simulink model "general_charger_2 (Jordans MacBook.lan's conflicted copy 2013-12-22)"  (R2013a)
settings: Solver=ode45  StartTime=0  StopTime=2.5  RelTol=1e-3
PreLoadFcn:
  | Ts =5e-6;
values from neighbouring files (symbols this model uses):
  ac_volt = 169    [charger_init.m]    (also in charger_init_simpl.m)
  Cdc = 2e-3    (= 0.002)    [charger_init.m]    (also in charger_init_simpl.m)
  dcAd = dcinvexp*(eye(dcnstates) + (Ts/2)*dcAc)    [charger_init.m]    (also in charger_init_simpl.m)
  dcBd = dcinvexp*dcBc    [charger_init.m]    (also in charger_init_simpl.m)
  dcCd = dcCc*dcinvexp*Ts    [charger_init.m]    (also in charger_init_simpl.m)
  dcDd = dcCc*dcinvexp*dcBc*(Ts/2) + dcDc    [charger_init.m]    (also in charger_init_simpl.m)
  Lin = 1.5e-3    (= 0.0015)    [charger_init.m]    (also in charger_init_simpl.m = 0.001)
  P = 1.92e3    (= 1920)    [charger_init.m]    (also in charger_init_simpl.m)
  Q = 0    [charger_init.m]    (also in charger_init_simpl.m)
  ramp = (dc_volt - Vdcmin)/(acdc_ramp_end_time)    (= 202)    [charger_init.m]    (also in charger_init_simpl.m = (dc_volt - Vdcmin)/(acdc_ramp_end_time))
  switch_Ts = 5e-5    (= 5e-05)    [charger_init.m]    (also in charger_init_simpl.m)
  sys_Ts = 5e-6    (= 5e-06)    [charger_init.m]    (also in charger_init_simpl.m)
  Vdcmin = ac_volt + 10    (= 179)    [charger_init.m]    (also in charger_init_simpl.m)
  voc = 105    [charger_init.m]    (also in charger_init_simpl.m)
undefined symbols (not defined in the file or in its folder): CESR, DiscIntNeverNeededParam, Rin
undefined symbols (not defined in the file): active_power_on, Ad, Bd, Cd, dc_volt, dcdc_iki, dcdc_ikp, dcdc_on, dcdc_vki, dcdc_vkp, Dd, dq_id_ki, dq_id_kp, dq_iq_ki, dq_iq_kp, dq_vdc_ki, dq_vdc_kp, P_ki, P_kp, Q_ki, Q_kp, reactive_power_on
libraries: simulink_extras x165, powerlib x52, simulink x29, powerlib_meascontrol x6
(part 6 of 6)

== system general_charger_2 (Jordans MacBook.lan's conflicted copy 2013-12-22)/control_stage/AC//DC Control/DQ Controller/discrete low pass filter1/q rounder9 ==
  in : Inport
  Gain9 : Gain  Gain=2^-q
  Idealized ADC quantizer : simulink_extras/Additional Discrete/Idealized ADC quantizer  NumberOfConverterBits=32  Vmin=-range  Vmax=range  OutputDataType=double  OutputNegativeValues=on
  out : Outport
  wires:
  in/1 -> Idealized ADC quantizer/1
  Idealized ADC quantizer/1 -> Gain9/1
  Gain9/1 -> out/1

== system general_charger_2 (Jordans MacBook.lan's conflicted copy 2013-12-22)/control_stage/AC//DC Control/PR Controller/Source Voltage PLL/AB->DQ ==
  A : Inport
  wt : Inport  Port=2
  Add1 : Sum  Inputs=-+
  Add2 : Sum
  Delay : Delay  DelayLength=round(1/f/4/Ts)  SampleTime=Ts
  Product{1..4} (4 alike) : Product  RndMeth=Zero
  Trigonometric Function : Trigonometry
  Trigonometric Function1 : Trigonometry  Operator=cos
  D : Outport
  Q : Outport  Port=2
  wires:
  Add2/1 -> D/1  "Vd"
  Trigonometric Function/1 -> Product2/1, Product1/1
  Product1/1 -> Add2/2
  Product4/1 -> Add2/1
  wt/1 -> Trigonometric Function1/1, Trigonometric Function/1
  Delay/1 -> Product1/2, Product3/2
  Product2/1 -> Add1/1
  Product3/1 -> Add1/2
  Add1/1 -> Q/1
  A/1 -> Delay/1, Product4/1, Product2/2
  Trigonometric Function1/1 -> Product3/1, Product4/2

== system general_charger_2 (Jordans MacBook.lan's conflicted copy 2013-12-22)/control_stage/AC//DC Control/PR Controller/Source Voltage PLL/PI2 ==
  in : Inport
  Add1 : Sum
  Add2 : Sum
  Ki : Gain  Gain=ki
  Kp : Gain  Gain=kp
  Tappe : simulink/Discrete/Tapped Delay  vinit=0.0  samptime=Ts_pi  NumDelays=1  DelayOrder=Oldest  includeCurrent=off
  Ts : Gain  Gain=Ts_pi
  integral saturation : Saturate  UpperLimit=int_sat_up  LowerLimit=int_sat_low  SampleTime=Ts_pi
  pi controller saturation : Saturate  UpperLimit=pi_sat_up  LowerLimit=pi_sat_low  SampleTime=Ts_pi
  out : Outport
  wires:
  Ts/1 -> Ki/1
  in/1 -> Kp/1, Ts/1  "vdc_error"
  Add1/1 -> integral saturation/1  "vdc_int_pi"
  Kp/1 -> Add2/2  "vdc_kp_pi"
  pi controller saturation/1 -> out/1
  Tappe/1 -> Add1/1
  Add2/1 -> pi controller saturation/1  "vdc_pi"
  Ki/1 -> Add1/2
  integral saturation/1 -> Add2/1, Tappe/1

== system general_charger_2 (Jordans MacBook.lan's conflicted copy 2013-12-22)/Measurements/Power and angle calculations/AB-DQ Transform/Vab_dq/AB->DQ/Vd Discretization Error Correction ==
  A : Inport
  wt : Inport  Port=2
  D : Inport  Port=3
  Add1 : Sum  Inputs=-+
  Add2 : Sum  Inputs=-+
  Gain2 : Gain  Gain=0.000078956
  Gain3 : Gain  Gain=0.012566039
  Product : Product
  Product1 : Product
  Product2 : Product
  Trigonometric Function : Trigonometry
  Trigonometric Function1 : Trigonometry
  Trigonometric Function2 : Trigonometry
  Trigonometric Function3 : Trigonometry  Operator=cos
  Vd_corr : Outport
  wires:
  Add1/1 -> Product2/2
  Add2/1 -> Vd_corr/1
  A/1 -> Product2/1
  wt/1 -> Trigonometric Function2/1, Trigonometric Function3/1, Trigonometric Function/1, Trigonometric Function1/1
  Trigonometric Function/1 -> Product/2
  Trigonometric Function3/1 -> Product1/2
  Product1/1 -> Gain3/1
  Product2/1 -> Add2/1
  Trigonometric Function1/1 -> Product/1
  Product/1 -> Gain2/1
  D/1 -> Add2/2
  Gain3/1 -> Add1/1
  Trigonometric Function2/1 -> Product1/1
  Gain2/1 -> Add1/2

== system general_charger_2 (Jordans MacBook.lan's conflicted copy 2013-12-22)/Measurements/Power and angle calculations/AB-DQ Transform/Vab_dq/AB->DQ/Vq Discretization Error Correction ==
  Q : Inport
  wt : Inport  Port=2
  A : Inport  Port=3
  Add1 : Sum  Inputs=-+
  Add2 : Sum
  Gain2 : Gain  Gain=0.000078956
  Gain3 : Gain  Gain=-0.012566039
  Product : Product
  Product1 : Product
  Product3 : Product
  Trigonometric Function : Trigonometry  Operator=cos
  Trigonometric Function1 : Trigonometry  Operator=cos
  Trigonometric Function2 : Trigonometry
  Trigonometric Function3 : Trigonometry  Operator=cos
  Vq_corr : Outport
  wires:
  wt/1 -> Trigonometric Function2/1, Trigonometric Function/1, Trigonometric Function1/1, Trigonometric Function3/1
  Trigonometric Function2/1 -> Product1/1
  Trigonometric Function3/1 -> Product1/2
  Product1/1 -> Gain2/1
  Trigonometric Function1/1 -> Product3/1
  Trigonometric Function/1 -> Product3/2
  Product3/1 -> Gain3/1
  Gain2/1 -> Add2/1
  Gain3/1 -> Add2/2
  Add2/1 -> Product/2
  A/1 -> Product/1
  Product/1 -> Add1/1
  Q/1 -> Add1/2
  Add1/1 -> Vq_corr/1

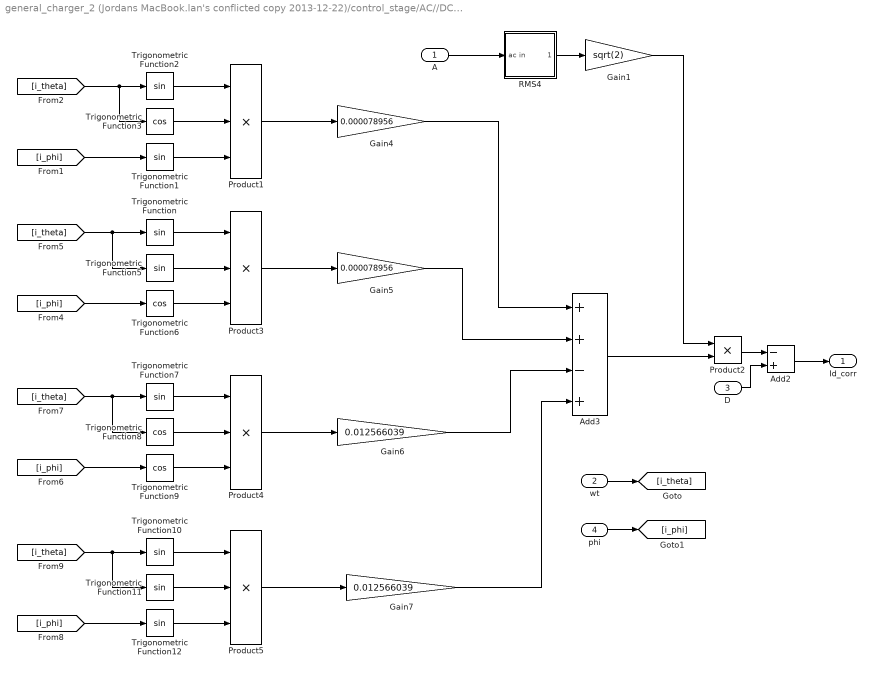
== system general_charger_2 (Jordans MacBook.lan's conflicted copy 2013-12-22)/control_stage/AC//DC Control/DQ Controller/AB-DQ Transform/AB->DQ/Id Discretization Error Correction ==
  A : Inport
  wt : Inport  Port=2
  D : Inport  Port=3
  phi : Inport  Port=4
  Add2 : Sum  Inputs=-+
  Add3 : Sum  Inputs=++-+
  Gain1 : Gain  Gain=sqrt(2)
  Gain4 : Gain  Gain=0.000078956
  Gain5 : Gain  Gain=0.000078956
  Gain6 : Gain  Gain=0.012566039
  Gain7 : Gain  Gain=0.012566039
  Product{1,3..5} (4 alike) : Product  Inputs=3
  Product2 : Product
  RMS4 : Subsystem  mask{f=60, rms_Ts=4e-4}
      mask prompts: f "Fundamental Frequency"; rms_Ts "Sample Time"
      mask init:
      | SpC=1/f/rms_Ts;
      | RSpC=ceil(SpC);
      | Delay=RSpC*rms_Ts;
      | Corr1=(SpC-RSpC)/2;
      | Corr2=(SpC-RSpC)/SpC;
      | K1=Corr1*Corr2;
      | K2=Corr2 + Corr1*Corr2;
      mask Display: disp('RMS')
  Trigonometric Function{,1..2,5,7,10..12} (8 alike) : Trigonometry
  Trigonometric Function{3,6,8..9} (4 alike) : Trigonometry  Operator=cos
  Id_corr : Outport
  wires:
  Add2/1 -> Id_corr/1
  Product2/1 -> Add2/1
  D/1 -> Add2/2
  wt/1 -> [i_theta]
  phi/1 -> [i_phi]
  [i_theta] -> Trigonometric Function3/1, Trigonometric Function2/1
  [i_phi] -> Trigonometric Function1/1
  Trigonometric Function1/1 -> Product1/3
  Trigonometric Function2/1 -> Product1/1
  Trigonometric Function3/1 -> Product1/2
  Product1/1 -> Gain4/1
  [i_theta] -> Trigonometric Function5/1, Trigonometric Function/1
  [i_phi] -> Trigonometric Function6/1
  Trigonometric Function5/1 -> Product3/2
  Trigonometric Function/1 -> Product3/1
  Trigonometric Function6/1 -> Product3/3
  [i_theta] -> Trigonometric Function8/1, Trigonometric Function7/1
  [i_phi] -> Trigonometric Function9/1
  Trigonometric Function8/1 -> Product4/2
  Trigonometric Function7/1 -> Product4/1
  Trigonometric Function9/1 -> Product4/3
  [i_theta] -> Trigonometric Function11/1, Trigonometric Function10/1
  [i_phi] -> Trigonometric Function12/1
  Trigonometric Function11/1 -> Product5/2
  Trigonometric Function10/1 -> Product5/1
  Trigonometric Function12/1 -> Product5/3
  Product3/1 -> Gain5/1
  Product4/1 -> Gain6/1
  Product5/1 -> Gain7/1
  Gain4/1 -> Add3/1
  Gain5/1 -> Add3/2
  Gain6/1 -> Add3/3
  Gain7/1 -> Add3/4
  Add3/1 -> Product2/2
  Gain1/1 -> Product2/1
  RMS4/1(rms out) -> Gain1/1
  A/1 -> RMS4/1(ac in)

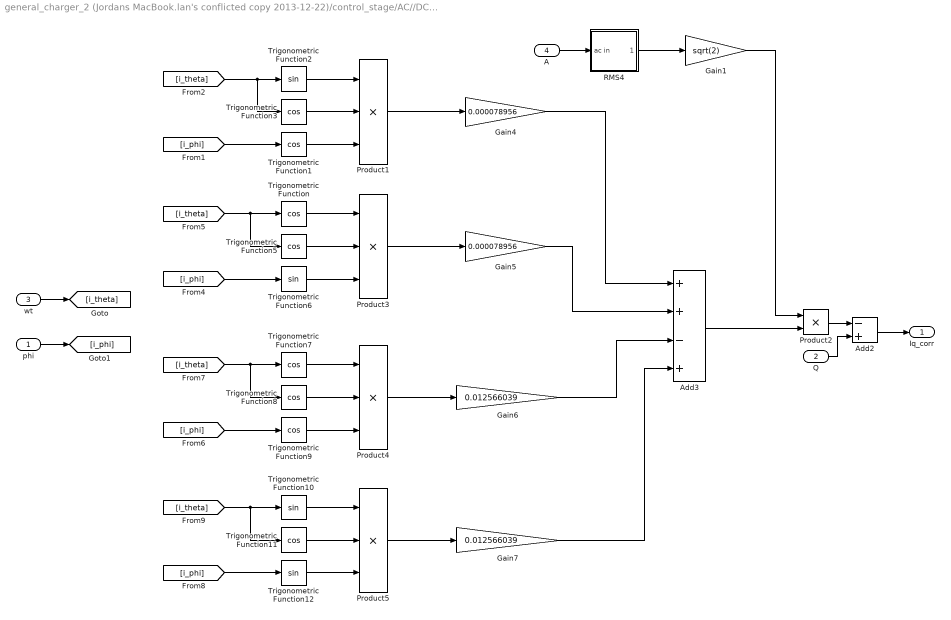
== system general_charger_2 (Jordans MacBook.lan's conflicted copy 2013-12-22)/control_stage/AC//DC Control/DQ Controller/AB-DQ Transform/AB->DQ/Iq Discretization Error Correction ==
  phi : Inport
  Q : Inport  Port=2
  wt : Inport  Port=3
  A : Inport  Port=4
  Add2 : Sum  Inputs=-+
  Add3 : Sum  Inputs=++-+
  Gain1 : Gain  Gain=sqrt(2)
  Gain4 : Gain  Gain=0.000078956
  Gain5 : Gain  Gain=0.000078956
  Gain6 : Gain  Gain=0.012566039
  Gain7 : Gain  Gain=0.012566039
  Product{1,3..5} (4 alike) : Product  Inputs=3
  Product2 : Product
  RMS4 : Subsystem  mask{f=60, rms_Ts=4e-4}
      mask prompts: f "Fundamental Frequency"; rms_Ts "Sample Time"
      mask init:
      | SpC=1/f/rms_Ts;
      | RSpC=ceil(SpC);
      | Delay=RSpC*rms_Ts;
      | Corr1=(SpC-RSpC)/2;
      | Corr2=(SpC-RSpC)/SpC;
      | K1=Corr1*Corr2;
      | K2=Corr2 + Corr1*Corr2;
      mask Display: disp('RMS')
  Trigonometric Function{,1,3,5,7..9,11} (8 alike) : Trigonometry  Operator=cos
  Trigonometric Function{2,6,10,12} (4 alike) : Trigonometry
  Iq_corr : Outport
  wires:
  Add2/1 -> Iq_corr/1
  Product2/1 -> Add2/1
  Q/1 -> Add2/2
  [i_theta] -> Trigonometric Function3/1, Trigonometric Function2/1
  [i_phi] -> Trigonometric Function1/1
  Trigonometric Function1/1 -> Product1/3
  Trigonometric Function2/1 -> Product1/1
  Trigonometric Function3/1 -> Product1/2
  Product1/1 -> Gain4/1
  [i_theta] -> Trigonometric Function5/1, Trigonometric Function/1
  [i_phi] -> Trigonometric Function6/1
  Trigonometric Function5/1 -> Product3/2
  Trigonometric Function/1 -> Product3/1
  Trigonometric Function6/1 -> Product3/3
  [i_theta] -> Trigonometric Function8/1, Trigonometric Function7/1
  [i_phi] -> Trigonometric Function9/1
  Trigonometric Function8/1 -> Product4/2
  Trigonometric Function7/1 -> Product4/1
  Trigonometric Function9/1 -> Product4/3
  [i_theta] -> Trigonometric Function11/1, Trigonometric Function10/1
  [i_phi] -> Trigonometric Function12/1
  Trigonometric Function11/1 -> Product5/2
  Trigonometric Function10/1 -> Product5/1
  Trigonometric Function12/1 -> Product5/3
  Product3/1 -> Gain5/1
  Product4/1 -> Gain6/1
  Product5/1 -> Gain7/1
  Gain4/1 -> Add3/1
  Gain5/1 -> Add3/2
  Gain6/1 -> Add3/3
  Gain7/1 -> Add3/4
  Add3/1 -> Product2/2
  Gain1/1 -> Product2/1
  wt/1 -> [i_theta]
  phi/1 -> [i_phi]
  RMS4/1(rms out) -> Gain1/1
  A/1 -> RMS4/1(ac in)

== system general_charger_2 (Jordans MacBook.lan's conflicted copy 2013-12-22)/control_stage/AC//DC Control/DQ Controller/AB-DQ Transform/PLL/AB->DQ ==
  A : Inport
  wt : Inport  Port=2
  Add1 : Sum  Inputs=-+
  Add2 : Sum
  Delay : Delay  DelayLength=RSpC  SampleTime=abdq_Ts
  Product{1..4} (4 alike) : Product  RndMeth=Zero
  Trigonometric Function : Trigonometry
  Trigonometric Function1 : Trigonometry  Operator=cos
  Vd Discretization Error Correction : Subsystem
  Vq Discretization Error Correction : Subsystem
  D : Outport
  Q : Outport  Port=2
  wires:
  Trigonometric Function/1 -> Product1/1, Product2/1
  Product1/1 -> Add2/2
  Product4/1 -> Add2/1
  Product2/1 -> Add1/1
  A/1 -> Vq Discretization Error Correction/3(A), Delay/1, Vd Discretization Error Correction/1(A), Product4/1, Product2/2
  Trigonometric Function1/1 -> Product4/2, Product3/1
  Product3/1 -> Add1/2
  Delay/1 -> Product1/2, Product3/2  "B"
  wt/1 -> [theta], Trigonometric Function1/1, Trigonometric Function/1
  Add2/1 -> Vd Discretization Error Correction/3(D)  "Vd"
  Add1/1 -> Vq Discretization Error Correction/1(Q)
  [theta] -> Vq Discretization Error Correction/2(wt)
  [theta] -> Vd Discretization Error Correction/2(wt)
  Vd Discretization Error Correction/1(Vd_corr) -> D/1
  Vq Discretization Error Correction/1(Vq_corr) -> Q/1

== system general_charger_2 (Jordans MacBook.lan's conflicted copy 2013-12-22)/control_stage/AC//DC Control/DQ Controller/AB-DQ Transform/PLL/PI1 ==
  in : Inport
  Add1 : Sum
  Add2 : Sum
  Ki : Gain  Gain=ki
  Kp : Gain  Gain=kp
  Tappe : simulink/Discrete/Tapped Delay  vinit=0.0  samptime=Ts_pi  NumDelays=1  DelayOrder=Oldest  includeCurrent=off
  Ts : Gain  Gain=Ts_pi
  integral saturation : Saturate  UpperLimit=int_sat_up  LowerLimit=int_sat_low  SampleTime=Ts_pi
  pi controller saturation : Saturate  UpperLimit=pi_sat_up  LowerLimit=pi_sat_low  SampleTime=Ts_pi
  out : Outport
  wires:
  Ts/1 -> Ki/1
  in/1 -> Kp/1, Ts/1  "vdc_error"
  Add1/1 -> integral saturation/1  "vdc_int_pi"
  Kp/1 -> Add2/2  "vdc_kp_pi"
  pi controller saturation/1 -> out/1
  Tappe/1 -> Add1/1
  Add2/1 -> pi controller saturation/1  "vdc_pi"
  Ki/1 -> Add1/2
  integral saturation/1 -> Add2/1, Tappe/1

== system general_charger_2 (Jordans MacBook.lan's conflicted copy 2013-12-22)/control_stage/AC//DC Control/DQ Controller/AB-DQ Transform/PLL/PI4 ==
  in : Inport
  Add1 : Sum
  Add2 : Sum
  Ki : Gain  Gain=ki
  Kp : Gain  Gain=kp
  Tappe : simulink/Discrete/Tapped Delay  vinit=0.0  samptime=Ts_pi  NumDelays=1  DelayOrder=Oldest  includeCurrent=off
  Ts : Gain  Gain=Ts_pi
  integral saturation : Saturate  UpperLimit=int_sat_up  LowerLimit=int_sat_low  SampleTime=Ts_pi
  pi controller saturation : Saturate  UpperLimit=pi_sat_up  LowerLimit=pi_sat_low  SampleTime=Ts_pi
  out : Outport
  wires:
  Ts/1 -> Ki/1
  in/1 -> Kp/1, Ts/1  "vdc_error"
  Add1/1 -> integral saturation/1  "vdc_int_pi"
  Kp/1 -> Add2/2  "vdc_kp_pi"
  pi controller saturation/1 -> out/1
  Tappe/1 -> Add1/1
  Add2/1 -> pi controller saturation/1  "vdc_pi"
  Ki/1 -> Add1/2
  integral saturation/1 -> Add2/1, Tappe/1

== system general_charger_2 (Jordans MacBook.lan's conflicted copy 2013-12-22)/control_stage/AC//DC Control/DQ Controller/DQ Controller Submodule/Reactive Power Control Module/PI4 ==
  in : Inport
  Add1 : Sum
  Add2 : Sum
  Ki : Gain  Gain=ki
  Kp : Gain  Gain=kp
  Tappe : simulink/Discrete/Tapped Delay  vinit=0.0  samptime=Ts_pi  NumDelays=1  DelayOrder=Oldest  includeCurrent=off
  Ts : Gain  Gain=Ts_pi
  integral saturation : Saturate  UpperLimit=int_sat_up  LowerLimit=int_sat_low  SampleTime=Ts_pi
  pi controller saturation : Saturate  UpperLimit=pi_sat_up  LowerLimit=pi_sat_low  SampleTime=Ts_pi
  out : Outport
  wires:
  Ts/1 -> Ki/1
  in/1 -> Kp/1, Ts/1  "vdc_error"
  Add1/1 -> integral saturation/1  "vdc_int_pi"
  Kp/1 -> Add2/2  "vdc_kp_pi"
  pi controller saturation/1 -> out/1
  Tappe/1 -> Add1/1
  Add2/1 -> pi controller saturation/1  "vdc_pi"
  Ki/1 -> Add1/2
  integral saturation/1 -> Add2/1, Tappe/1

== system general_charger_2 (Jordans MacBook.lan's conflicted copy 2013-12-22)/control_stage/AC//DC Control/DQ Controller/discrete low pass filter1/Ad(1,1)/q rounder16 ==
  in : Inport
  Gain9 : Gain  Gain=2^-q
  Idealized ADC quantizer : simulink_extras/Additional Discrete/Idealized ADC quantizer  NumberOfConverterBits=32  Vmin=-range  Vmax=range  OutputDataType=double  OutputNegativeValues=on
  out : Outport
  wires:
  in/1 -> Idealized ADC quantizer/1
  Idealized ADC quantizer/1 -> Gain9/1
  Gain9/1 -> out/1

== system general_charger_2 (Jordans MacBook.lan's conflicted copy 2013-12-22)/control_stage/AC//DC Control/DQ Controller/discrete low pass filter1/Ad(1,2)/q rounder16 ==
  in : Inport
  Gain9 : Gain  Gain=2^-q
  Idealized ADC quantizer : simulink_extras/Additional Discrete/Idealized ADC quantizer  NumberOfConverterBits=32  Vmin=-range  Vmax=range  OutputDataType=double  OutputNegativeValues=on
  out : Outport
  wires:
  in/1 -> Idealized ADC quantizer/1
  Idealized ADC quantizer/1 -> Gain9/1
  Gain9/1 -> out/1

== system general_charger_2 (Jordans MacBook.lan's conflicted copy 2013-12-22)/control_stage/AC//DC Control/DQ Controller/discrete low pass filter1/Ad(1,3)/q rounder16 ==
  in : Inport
  Gain9 : Gain  Gain=2^-q
  Idealized ADC quantizer : simulink_extras/Additional Discrete/Idealized ADC quantizer  NumberOfConverterBits=32  Vmin=-range  Vmax=range  OutputDataType=double  OutputNegativeValues=on
  out : Outport
  wires:
  in/1 -> Idealized ADC quantizer/1
  Idealized ADC quantizer/1 -> Gain9/1
  Gain9/1 -> out/1

== system general_charger_2 (Jordans MacBook.lan's conflicted copy 2013-12-22)/control_stage/AC//DC Control/DQ Controller/discrete low pass filter1/Ad(2,1)/q rounder16 ==
  in : Inport
  Gain9 : Gain  Gain=2^-q
  Idealized ADC quantizer : simulink_extras/Additional Discrete/Idealized ADC quantizer  NumberOfConverterBits=32  Vmin=-range  Vmax=range  OutputDataType=double  OutputNegativeValues=on
  out : Outport
  wires:
  in/1 -> Idealized ADC quantizer/1
  Idealized ADC quantizer/1 -> Gain9/1
  Gain9/1 -> out/1

== system general_charger_2 (Jordans MacBook.lan's conflicted copy 2013-12-22)/control_stage/AC//DC Control/DQ Controller/discrete low pass filter1/Ad(2,2)/q rounder16 ==
  in : Inport
  Gain9 : Gain  Gain=2^-q
  Idealized ADC quantizer : simulink_extras/Additional Discrete/Idealized ADC quantizer  NumberOfConverterBits=32  Vmin=-range  Vmax=range  OutputDataType=double  OutputNegativeValues=on
  out : Outport
  wires:
  in/1 -> Idealized ADC quantizer/1
  Idealized ADC quantizer/1 -> Gain9/1
  Gain9/1 -> out/1

== system general_charger_2 (Jordans MacBook.lan's conflicted copy 2013-12-22)/control_stage/AC//DC Control/DQ Controller/discrete low pass filter1/Ad(2,3)/q rounder16 ==
  in : Inport
  Gain9 : Gain  Gain=2^-q
  Idealized ADC quantizer : simulink_extras/Additional Discrete/Idealized ADC quantizer  NumberOfConverterBits=32  Vmin=-range  Vmax=range  OutputDataType=double  OutputNegativeValues=on
  out : Outport
  wires:
  in/1 -> Idealized ADC quantizer/1
  Idealized ADC quantizer/1 -> Gain9/1
  Gain9/1 -> out/1

== system general_charger_2 (Jordans MacBook.lan's conflicted copy 2013-12-22)/control_stage/AC//DC Control/DQ Controller/discrete low pass filter1/Ad(3,1)/q rounder16 ==
  in : Inport
  Gain9 : Gain  Gain=2^-q
  Idealized ADC quantizer : simulink_extras/Additional Discrete/Idealized ADC quantizer  NumberOfConverterBits=32  Vmin=-range  Vmax=range  OutputDataType=double  OutputNegativeValues=on
  out : Outport
  wires:
  in/1 -> Idealized ADC quantizer/1
  Idealized ADC quantizer/1 -> Gain9/1
  Gain9/1 -> out/1

== system general_charger_2 (Jordans MacBook.lan's conflicted copy 2013-12-22)/control_stage/AC//DC Control/DQ Controller/discrete low pass filter1/Ad(3,2)/q rounder16 ==
  in : Inport
  Gain9 : Gain  Gain=2^-q
  Idealized ADC quantizer : simulink_extras/Additional Discrete/Idealized ADC quantizer  NumberOfConverterBits=32  Vmin=-range  Vmax=range  OutputDataType=double  OutputNegativeValues=on
  out : Outport
  wires:
  in/1 -> Idealized ADC quantizer/1
  Idealized ADC quantizer/1 -> Gain9/1
  Gain9/1 -> out/1

== system general_charger_2 (Jordans MacBook.lan's conflicted copy 2013-12-22)/control_stage/AC//DC Control/DQ Controller/discrete low pass filter1/Ad(3,3)/q rounder16 ==
  in : Inport
  Gain9 : Gain  Gain=2^-q
  Idealized ADC quantizer : simulink_extras/Additional Discrete/Idealized ADC quantizer  NumberOfConverterBits=32  Vmin=-range  Vmax=range  OutputDataType=double  OutputNegativeValues=on
  out : Outport
  wires:
  in/1 -> Idealized ADC quantizer/1
  Idealized ADC quantizer/1 -> Gain9/1
  Gain9/1 -> out/1

== system general_charger_2 (Jordans MacBook.lan's conflicted copy 2013-12-22)/control_stage/AC//DC Control/DQ Controller/discrete low pass filter1/Bd(1)/q rounder16 ==
  in : Inport
  Gain9 : Gain  Gain=2^-q
  Idealized ADC quantizer : simulink_extras/Additional Discrete/Idealized ADC quantizer  NumberOfConverterBits=32  Vmin=-range  Vmax=range  OutputDataType=double  OutputNegativeValues=on
  out : Outport
  wires:
  in/1 -> Idealized ADC quantizer/1
  Idealized ADC quantizer/1 -> Gain9/1
  Gain9/1 -> out/1

== system general_charger_2 (Jordans MacBook.lan's conflicted copy 2013-12-22)/control_stage/AC//DC Control/DQ Controller/discrete low pass filter1/Bd(2)/q rounder16 ==
  in : Inport
  Gain9 : Gain  Gain=2^-q
  Idealized ADC quantizer : simulink_extras/Additional Discrete/Idealized ADC quantizer  NumberOfConverterBits=32  Vmin=-range  Vmax=range  OutputDataType=double  OutputNegativeValues=on
  out : Outport
  wires:
  in/1 -> Idealized ADC quantizer/1
  Idealized ADC quantizer/1 -> Gain9/1
  Gain9/1 -> out/1

== system general_charger_2 (Jordans MacBook.lan's conflicted copy 2013-12-22)/control_stage/AC//DC Control/DQ Controller/discrete low pass filter1/Bd(3)/q rounder16 ==
  in : Inport
  Gain9 : Gain  Gain=2^-q
  Idealized ADC quantizer : simulink_extras/Additional Discrete/Idealized ADC quantizer  NumberOfConverterBits=32  Vmin=-range  Vmax=range  OutputDataType=double  OutputNegativeValues=on
  out : Outport
  wires:
  in/1 -> Idealized ADC quantizer/1
  Idealized ADC quantizer/1 -> Gain9/1
  Gain9/1 -> out/1

== system general_charger_2 (Jordans MacBook.lan's conflicted copy 2013-12-22)/control_stage/AC//DC Control/DQ Controller/discrete low pass filter1/Cd(1)/q rounder16 ==
  in : Inport
  Gain9 : Gain  Gain=2^-q
  Idealized ADC quantizer : simulink_extras/Additional Discrete/Idealized ADC quantizer  NumberOfConverterBits=32  Vmin=-range  Vmax=range  OutputDataType=double  OutputNegativeValues=on
  out : Outport
  wires:
  in/1 -> Idealized ADC quantizer/1
  Idealized ADC quantizer/1 -> Gain9/1
  Gain9/1 -> out/1

== system general_charger_2 (Jordans MacBook.lan's conflicted copy 2013-12-22)/control_stage/AC//DC Control/DQ Controller/discrete low pass filter1/Cd(2)/q rounder16 ==
  in : Inport
  Gain9 : Gain  Gain=2^-q
  Idealized ADC quantizer : simulink_extras/Additional Discrete/Idealized ADC quantizer  NumberOfConverterBits=32  Vmin=-range  Vmax=range  OutputDataType=double  OutputNegativeValues=on
  out : Outport
  wires:
  in/1 -> Idealized ADC quantizer/1
  Idealized ADC quantizer/1 -> Gain9/1
  Gain9/1 -> out/1

== system general_charger_2 (Jordans MacBook.lan's conflicted copy 2013-12-22)/control_stage/AC//DC Control/DQ Controller/discrete low pass filter1/Cd(3)/q rounder16 ==
  in : Inport
  Gain9 : Gain  Gain=2^-q
  Idealized ADC quantizer : simulink_extras/Additional Discrete/Idealized ADC quantizer  NumberOfConverterBits=32  Vmin=-range  Vmax=range  OutputDataType=double  OutputNegativeValues=on
  out : Outport
  wires:
  in/1 -> Idealized ADC quantizer/1
  Idealized ADC quantizer/1 -> Gain9/1
  Gain9/1 -> out/1

== system general_charger_2 (Jordans MacBook.lan's conflicted copy 2013-12-22)/control_stage/AC//DC Control/DQ Controller/discrete low pass filter1/Dd/q rounder16 ==
  in : Inport
  Gain9 : Gain  Gain=2^-q
  Idealized ADC quantizer : simulink_extras/Additional Discrete/Idealized ADC quantizer  NumberOfConverterBits=32  Vmin=-range  Vmax=range  OutputDataType=double  OutputNegativeValues=on
  out : Outport
  wires:
  in/1 -> Idealized ADC quantizer/1
  Idealized ADC quantizer/1 -> Gain9/1
  Gain9/1 -> out/1

== system general_charger_2 (Jordans MacBook.lan's conflicted copy 2013-12-22)/control_stage/AC//DC Control/DQ Controller/AB-DQ Transform/AB->DQ/Id Discretization Error Correction/RMS4 ==
  ac in : Inport
  Constant : Constant  Value=K1
  Constant1 : Constant  Value=f  SampleTime=-1
  Constant2 : Constant  Value=K2
  Delay : Delay  DelayLength=ceil(SpC)  SampleTime=rms_Ts
  Gain : Gain  Gain=K1  SaturateOnIntegerOverflow=on  OutDataTypeStr=Inherit: Same as input  ParamDataTypeStr=Inherit: Same as input
  Gain1 : Gain  Gain=K2  SaturateOnIntegerOverflow=on  OutDataTypeStr=Inherit: Same as input  ParamDataTypeStr=Inherit: Same as input
  PI3 : Subsystem  mask{ki=1, kp=0, Ts_pi=rms_Ts, int_sat_up=inf, int_sat_low=-inf, pi_sat_up=inf, pi_sat_low=-inf}
      mask prompts: ki "Integral Gain"; kp "Proportional Gain"; Ts_pi "Sample Time"; int_sat_up "Integral Saturation Upper"; int_sat_low "Integral Saturation Lower"; pi_sat_up "PI Controller Saturation Upper"; pi_sat_low "PI Controller Saturation Lower"
      mask Display: disp('PI')
  Product3 : Product  SaturateOnIntegerOverflow=on  InputSameDT=on  OutDataTypeStr=Inherit: Same as first input
  Product4 : Product  SaturateOnIntegerOverflow=on  InputSameDT=on  OutDataTypeStr=Inherit: Same as first input
  Pulse Generator : DiscretePulseGenerator  Period=rms_Ts/sys_Ts  SampleTime=sys_Ts
  Sample and Hold : powerlib_meascontrol/Additional Components/Sample and Hold  ic=0  Ts=sys_Ts
  Saturation : Saturate  UpperLimit=inf  LowerLimit=0
  Scope : Scope  NumInputPorts=2
      settings: YMin=-5~-5  YMax=5~5  SaveName=ScopeData2
  Sqrt : Sqrt  SaturateOnIntegerOverflow=on
  Sum1 : Sum  Inputs=+-  SaturateOnIntegerOverflow=on  InputSameDT=on  OutDataTypeStr=Inherit: Same as first input
  Sum2 : Sum  Inputs=-+  SaturateOnIntegerOverflow=on  InputSameDT=on  OutDataTypeStr=Inherit: Same as first input
  Sum3 : Sum  SaturateOnIntegerOverflow=on  InputSameDT=on  OutDataTypeStr=Inherit: Same as first input
  Unit Delay : UnitDelay  SampleTime=rms_Ts
  rms out : Outport
  wires:
  Sum2/1 -> Product4/1
  Constant1/1 -> Product4/2
  Delay/1 -> Sum2/1
  Product3/1 -> Unit Delay/1, Gain1/1, PI3/1(in)
  PI3/1(out) -> Sum2/2, Delay/1
  Sqrt/1 -> rms out/1
  Gain1/1 -> Sum1/1
  Unit Delay/1 -> Gain/1
  Gain/1 -> Sum1/2
  Product4/1 -> Sum3/1
  Sum3/1 -> Saturation/1
  Sum1/1 -> Sum3/2  "Correction"
  Saturation/1 -> Sqrt/1
  Pulse Generator/1 -> Sample and Hold/2
  Sample and Hold/1 -> Product3/1, Product3/2
  ac in/1 -> Sample and Hold/1
  Constant2/1 -> Scope/2
  Constant/1 -> Scope/1

== system general_charger_2 (Jordans MacBook.lan's conflicted copy 2013-12-22)/control_stage/AC//DC Control/DQ Controller/AB-DQ Transform/AB->DQ/Iq Discretization Error Correction/RMS4 ==
  ac in : Inport
  Constant : Constant  Value=K1
  Constant1 : Constant  Value=f  SampleTime=-1
  Constant2 : Constant  Value=K2
  Delay : Delay  DelayLength=ceil(SpC)  SampleTime=rms_Ts
  Gain : Gain  Gain=K1  SaturateOnIntegerOverflow=on  OutDataTypeStr=Inherit: Same as input  ParamDataTypeStr=Inherit: Same as input
  Gain1 : Gain  Gain=K2  SaturateOnIntegerOverflow=on  OutDataTypeStr=Inherit: Same as input  ParamDataTypeStr=Inherit: Same as input
  PI3 : Subsystem  mask{ki=1, kp=0, Ts_pi=rms_Ts, int_sat_up=inf, int_sat_low=-inf, pi_sat_up=inf, pi_sat_low=-inf}
      mask prompts: ki "Integral Gain"; kp "Proportional Gain"; Ts_pi "Sample Time"; int_sat_up "Integral Saturation Upper"; int_sat_low "Integral Saturation Lower"; pi_sat_up "PI Controller Saturation Upper"; pi_sat_low "PI Controller Saturation Lower"
      mask Display: disp('PI')
  Product3 : Product  SaturateOnIntegerOverflow=on  InputSameDT=on  OutDataTypeStr=Inherit: Same as first input
  Product4 : Product  SaturateOnIntegerOverflow=on  InputSameDT=on  OutDataTypeStr=Inherit: Same as first input
  Pulse Generator : DiscretePulseGenerator  Period=rms_Ts/sys_Ts  SampleTime=sys_Ts
  Sample and Hold : powerlib_meascontrol/Additional Components/Sample and Hold  ic=0  Ts=sys_Ts
  Saturation : Saturate  UpperLimit=inf  LowerLimit=0
  Scope : Scope  NumInputPorts=2
      settings: YMin=-5~-5  YMax=5~5  SaveName=ScopeData2
  Sqrt : Sqrt  SaturateOnIntegerOverflow=on
  Sum1 : Sum  Inputs=+-  SaturateOnIntegerOverflow=on  InputSameDT=on  OutDataTypeStr=Inherit: Same as first input
  Sum2 : Sum  Inputs=-+  SaturateOnIntegerOverflow=on  InputSameDT=on  OutDataTypeStr=Inherit: Same as first input
  Sum3 : Sum  SaturateOnIntegerOverflow=on  InputSameDT=on  OutDataTypeStr=Inherit: Same as first input
  Unit Delay : UnitDelay  SampleTime=rms_Ts
  rms out : Outport
  wires:
  Sum2/1 -> Product4/1
  Constant1/1 -> Product4/2
  Delay/1 -> Sum2/1
  Product3/1 -> Unit Delay/1, Gain1/1, PI3/1(in)
  PI3/1(out) -> Sum2/2, Delay/1
  Sqrt/1 -> rms out/1
  Gain1/1 -> Sum1/1
  Unit Delay/1 -> Gain/1
  Gain/1 -> Sum1/2
  Product4/1 -> Sum3/1
  Sum3/1 -> Saturation/1
  Sum1/1 -> Sum3/2  "Correction"
  Saturation/1 -> Sqrt/1
  Pulse Generator/1 -> Sample and Hold/2
  Sample and Hold/1 -> Product3/1, Product3/2
  ac in/1 -> Sample and Hold/1
  Constant2/1 -> Scope/2
  Constant/1 -> Scope/1

== system general_charger_2 (Jordans MacBook.lan's conflicted copy 2013-12-22)/control_stage/AC//DC Control/DQ Controller/AB-DQ Transform/PLL/AB->DQ/Vd Discretization Error Correction ==
  A : Inport
  wt : Inport  Port=2
  D : Inport  Port=3
  Add1 : Sum  Inputs=-+
  Add2 : Sum  Inputs=-+
  Gain1 : Gain  Gain=sqrt(2)
  Gain2 : Gain  Gain=0.000078956
  Gain3 : Gain  Gain=0.012566039
  Product : Product
  Product1 : Product
  Product2 : Product
  RMS4 : Subsystem  mask{f=60, rms_Ts=4e-4}
      mask prompts: f "Fundamental Frequency"; rms_Ts "Sample Time"
      mask init:
      | SpC=1/f/rms_Ts;
      | RSpC=ceil(SpC);
      | Delay=RSpC*rms_Ts;
      | Corr1=(SpC-RSpC)/2;
      | Corr2=(SpC-RSpC)/SpC;
      | K1=Corr1*Corr2;
      | K2=Corr2 + Corr1*Corr2;
      mask Display: disp('RMS')
  Trigonometric Function : Trigonometry
  Trigonometric Function1 : Trigonometry
  Trigonometric Function2 : Trigonometry
  Trigonometric Function3 : Trigonometry  Operator=cos
  Vd_corr : Outport
  wires:
  Add1/1 -> Product2/2
  Add2/1 -> Vd_corr/1
  A/1 -> RMS4/1(ac in)
  wt/1 -> Trigonometric Function2/1, Trigonometric Function3/1, Trigonometric Function/1, Trigonometric Function1/1
  Trigonometric Function/1 -> Product/2
  Trigonometric Function3/1 -> Product1/2
  RMS4/1(rms out) -> Gain1/1
  Product1/1 -> Gain3/1
  Product2/1 -> Add2/1
  Trigonometric Function1/1 -> Product/1
  Gain1/1 -> Product2/1
  Product/1 -> Gain2/1
  D/1 -> Add2/2
  Gain3/1 -> Add1/1
  Trigonometric Function2/1 -> Product1/1
  Gain2/1 -> Add1/2

== system general_charger_2 (Jordans MacBook.lan's conflicted copy 2013-12-22)/control_stage/AC//DC Control/DQ Controller/AB-DQ Transform/PLL/AB->DQ/Vq Discretization Error Correction ==
  Q : Inport
  wt : Inport  Port=2
  A : Inport  Port=3
  Add1 : Sum  Inputs=-+
  Add2 : Sum
  Gain1 : Gain  Gain=sqrt(2)
  Gain2 : Gain  Gain=0.000078956
  Gain3 : Gain  Gain=-0.012566039
  Product : Product
  Product1 : Product
  Product3 : Product
  RMS4 : Subsystem  mask{f=60, rms_Ts=4e-4}
      mask prompts: f "Fundamental Frequency"; rms_Ts "Sample Time"
      mask init:
      | SpC=1/f/rms_Ts;
      | RSpC=ceil(SpC);
      | Delay=RSpC*rms_Ts;
      | Corr1=(SpC-RSpC)/2;
      | Corr2=(SpC-RSpC)/SpC;
      | K1=Corr1*Corr2;
      | K2=Corr2 + Corr1*Corr2;
      mask Display: disp('RMS')
  Trigonometric Function : Trigonometry  Operator=cos
  Trigonometric Function1 : Trigonometry  Operator=cos
  Trigonometric Function2 : Trigonometry
  Trigonometric Function3 : Trigonometry  Operator=cos
  Vq_corr : Outport
  wires:
  A/1 -> RMS4/1(ac in)
  RMS4/1(rms out) -> Gain1/1
  wt/1 -> Trigonometric Function2/1, Trigonometric Function3/1, Trigonometric Function/1, Trigonometric Function1/1
  Trigonometric Function2/1 -> Product1/1
  Trigonometric Function3/1 -> Product1/2
  Product1/1 -> Gain2/1
  Trigonometric Function1/1 -> Product3/1
  Trigonometric Function/1 -> Product3/2
  Product3/1 -> Gain3/1
  Gain2/1 -> Add2/1
  Gain3/1 -> Add2/2
  Add2/1 -> Product/2
  Gain1/1 -> Product/1
  Product/1 -> Add1/1
  Q/1 -> Add1/2
  Add1/1 -> Vq_corr/1

== system general_charger_2 (Jordans MacBook.lan's conflicted copy 2013-12-22)/control_stage/AC//DC Control/DQ Controller/AB-DQ Transform/AB->DQ/Id Discretization Error Correction/RMS4/PI3 ==
  in : Inport
  Add1 : Sum
  Add2 : Sum
  Ki : Gain  Gain=ki
  Kp : Gain  Gain=kp
  Tappe : simulink/Discrete/Tapped Delay  vinit=0.0  samptime=Ts_pi  NumDelays=1  DelayOrder=Oldest  includeCurrent=off
  Ts : Gain  Gain=Ts_pi
  integral saturation : Saturate  UpperLimit=int_sat_up  LowerLimit=int_sat_low  SampleTime=Ts_pi
  pi controller saturation : Saturate  UpperLimit=pi_sat_up  LowerLimit=pi_sat_low  SampleTime=Ts_pi
  out : Outport
  wires:
  Ts/1 -> Ki/1
  in/1 -> Kp/1, Ts/1  "vdc_error"
  Add1/1 -> integral saturation/1  "vdc_int_pi"
  Kp/1 -> Add2/2  "vdc_kp_pi"
  pi controller saturation/1 -> out/1
  Tappe/1 -> Add1/1
  Add2/1 -> pi controller saturation/1  "vdc_pi"
  Ki/1 -> Add1/2
  integral saturation/1 -> Add2/1, Tappe/1

== system general_charger_2 (Jordans MacBook.lan's conflicted copy 2013-12-22)/control_stage/AC//DC Control/DQ Controller/AB-DQ Transform/AB->DQ/Iq Discretization Error Correction/RMS4/PI3 ==
  in : Inport
  Add1 : Sum
  Add2 : Sum
  Ki : Gain  Gain=ki
  Kp : Gain  Gain=kp
  Tappe : simulink/Discrete/Tapped Delay  vinit=0.0  samptime=Ts_pi  NumDelays=1  DelayOrder=Oldest  includeCurrent=off
  Ts : Gain  Gain=Ts_pi
  integral saturation : Saturate  UpperLimit=int_sat_up  LowerLimit=int_sat_low  SampleTime=Ts_pi
  pi controller saturation : Saturate  UpperLimit=pi_sat_up  LowerLimit=pi_sat_low  SampleTime=Ts_pi
  out : Outport
  wires:
  Ts/1 -> Ki/1
  in/1 -> Kp/1, Ts/1  "vdc_error"
  Add1/1 -> integral saturation/1  "vdc_int_pi"
  Kp/1 -> Add2/2  "vdc_kp_pi"
  pi controller saturation/1 -> out/1
  Tappe/1 -> Add1/1
  Add2/1 -> pi controller saturation/1  "vdc_pi"
  Ki/1 -> Add1/2
  integral saturation/1 -> Add2/1, Tappe/1

== system general_charger_2 (Jordans MacBook.lan's conflicted copy 2013-12-22)/control_stage/AC//DC Control/DQ Controller/AB-DQ Transform/PLL/AB->DQ/Vd Discretization Error Correction/RMS4 ==
  ac in : Inport
  Constant : Constant  Value=K1
  Constant1 : Constant  Value=f  SampleTime=-1
  Constant2 : Constant  Value=K2
  Delay : Delay  DelayLength=ceil(SpC)  SampleTime=rms_Ts
  Gain : Gain  Gain=K1  SaturateOnIntegerOverflow=on  OutDataTypeStr=Inherit: Same as input  ParamDataTypeStr=Inherit: Same as input
  Gain1 : Gain  Gain=K2  SaturateOnIntegerOverflow=on  OutDataTypeStr=Inherit: Same as input  ParamDataTypeStr=Inherit: Same as input
  PI3 : Subsystem  mask{ki=1, kp=0, Ts_pi=rms_Ts, int_sat_up=inf, int_sat_low=-inf, pi_sat_up=inf, pi_sat_low=-inf}
      mask prompts: ki "Integral Gain"; kp "Proportional Gain"; Ts_pi "Sample Time"; int_sat_up "Integral Saturation Upper"; int_sat_low "Integral Saturation Lower"; pi_sat_up "PI Controller Saturation Upper"; pi_sat_low "PI Controller Saturation Lower"
      mask Display: disp('PI')
  Product3 : Product  SaturateOnIntegerOverflow=on  InputSameDT=on  OutDataTypeStr=Inherit: Same as first input
  Product4 : Product  SaturateOnIntegerOverflow=on  InputSameDT=on  OutDataTypeStr=Inherit: Same as first input
  Pulse Generator : DiscretePulseGenerator  Period=rms_Ts/sys_Ts  SampleTime=sys_Ts
  Sample and Hold : powerlib_meascontrol/Additional Components/Sample and Hold  ic=0  Ts=sys_Ts
  Saturation : Saturate  UpperLimit=inf  LowerLimit=0
  Scope : Scope  NumInputPorts=2
      settings: YMin=-5~-5  YMax=5~5  SaveName=ScopeData2
  Sqrt : Sqrt  SaturateOnIntegerOverflow=on
  Sum1 : Sum  Inputs=+-  SaturateOnIntegerOverflow=on  InputSameDT=on  OutDataTypeStr=Inherit: Same as first input
  Sum2 : Sum  Inputs=-+  SaturateOnIntegerOverflow=on  InputSameDT=on  OutDataTypeStr=Inherit: Same as first input
  Sum3 : Sum  SaturateOnIntegerOverflow=on  InputSameDT=on  OutDataTypeStr=Inherit: Same as first input
  Unit Delay : UnitDelay  SampleTime=rms_Ts
  rms out : Outport
  wires:
  Sum2/1 -> Product4/1
  Constant1/1 -> Product4/2
  Delay/1 -> Sum2/1
  Product3/1 -> Unit Delay/1, Gain1/1, PI3/1(in)
  PI3/1(out) -> Sum2/2, Delay/1
  Sqrt/1 -> rms out/1
  Gain1/1 -> Sum1/1
  Unit Delay/1 -> Gain/1
  Gain/1 -> Sum1/2
  Product4/1 -> Sum3/1
  Sum3/1 -> Saturation/1
  Sum1/1 -> Sum3/2  "Correction"
  Saturation/1 -> Sqrt/1
  Pulse Generator/1 -> Sample and Hold/2
  Sample and Hold/1 -> Product3/1, Product3/2
  ac in/1 -> Sample and Hold/1
  Constant2/1 -> Scope/2
  Constant/1 -> Scope/1

== system general_charger_2 (Jordans MacBook.lan's conflicted copy 2013-12-22)/control_stage/AC//DC Control/DQ Controller/AB-DQ Transform/PLL/AB->DQ/Vq Discretization Error Correction/RMS4 ==
  ac in : Inport
  Constant : Constant  Value=K1
  Constant1 : Constant  Value=f  SampleTime=-1
  Constant2 : Constant  Value=K2
  Delay : Delay  DelayLength=ceil(SpC)  SampleTime=rms_Ts
  Gain : Gain  Gain=K1  SaturateOnIntegerOverflow=on  OutDataTypeStr=Inherit: Same as input  ParamDataTypeStr=Inherit: Same as input
  Gain1 : Gain  Gain=K2  SaturateOnIntegerOverflow=on  OutDataTypeStr=Inherit: Same as input  ParamDataTypeStr=Inherit: Same as input
  PI3 : Subsystem  mask{ki=1, kp=0, Ts_pi=rms_Ts, int_sat_up=inf, int_sat_low=-inf, pi_sat_up=inf, pi_sat_low=-inf}
      mask prompts: ki "Integral Gain"; kp "Proportional Gain"; Ts_pi "Sample Time"; int_sat_up "Integral Saturation Upper"; int_sat_low "Integral Saturation Lower"; pi_sat_up "PI Controller Saturation Upper"; pi_sat_low "PI Controller Saturation Lower"
      mask Display: disp('PI')
  Product3 : Product  SaturateOnIntegerOverflow=on  InputSameDT=on  OutDataTypeStr=Inherit: Same as first input
  Product4 : Product  SaturateOnIntegerOverflow=on  InputSameDT=on  OutDataTypeStr=Inherit: Same as first input
  Pulse Generator : DiscretePulseGenerator  Period=rms_Ts/sys_Ts  SampleTime=sys_Ts
  Sample and Hold : powerlib_meascontrol/Additional Components/Sample and Hold  ic=0  Ts=sys_Ts
  Saturation : Saturate  UpperLimit=inf  LowerLimit=0
  Scope : Scope  NumInputPorts=2
      settings: YMin=-5~-5  YMax=5~5  SaveName=ScopeData2
  Sqrt : Sqrt  SaturateOnIntegerOverflow=on
  Sum1 : Sum  Inputs=+-  SaturateOnIntegerOverflow=on  InputSameDT=on  OutDataTypeStr=Inherit: Same as first input
  Sum2 : Sum  Inputs=-+  SaturateOnIntegerOverflow=on  InputSameDT=on  OutDataTypeStr=Inherit: Same as first input
  Sum3 : Sum  SaturateOnIntegerOverflow=on  InputSameDT=on  OutDataTypeStr=Inherit: Same as first input
  Unit Delay : UnitDelay  SampleTime=rms_Ts
  rms out : Outport
  wires:
  Sum2/1 -> Product4/1
  Constant1/1 -> Product4/2
  Delay/1 -> Sum2/1
  Product3/1 -> Unit Delay/1, Gain1/1, PI3/1(in)
  PI3/1(out) -> Sum2/2, Delay/1
  Sqrt/1 -> rms out/1
  Gain1/1 -> Sum1/1
  Unit Delay/1 -> Gain/1
  Gain/1 -> Sum1/2
  Product4/1 -> Sum3/1
  Sum3/1 -> Saturation/1
  Sum1/1 -> Sum3/2  "Correction"
  Saturation/1 -> Sqrt/1
  Pulse Generator/1 -> Sample and Hold/2
  Sample and Hold/1 -> Product3/1, Product3/2
  ac in/1 -> Sample and Hold/1
  Constant2/1 -> Scope/2
  Constant/1 -> Scope/1

== system general_charger_2 (Jordans MacBook.lan's conflicted copy 2013-12-22)/control_stage/AC//DC Control/DQ Controller/AB-DQ Transform/PLL/AB->DQ/Vd Discretization Error Correction/RMS4/PI3 ==
  in : Inport
  Add1 : Sum
  Add2 : Sum
  Ki : Gain  Gain=ki
  Kp : Gain  Gain=kp
  Tappe : simulink/Discrete/Tapped Delay  vinit=0.0  samptime=Ts_pi  NumDelays=1  DelayOrder=Oldest  includeCurrent=off
  Ts : Gain  Gain=Ts_pi
  integral saturation : Saturate  UpperLimit=int_sat_up  LowerLimit=int_sat_low  SampleTime=Ts_pi
  pi controller saturation : Saturate  UpperLimit=pi_sat_up  LowerLimit=pi_sat_low  SampleTime=Ts_pi
  out : Outport
  wires:
  Ts/1 -> Ki/1
  in/1 -> Kp/1, Ts/1  "vdc_error"
  Add1/1 -> integral saturation/1  "vdc_int_pi"
  Kp/1 -> Add2/2  "vdc_kp_pi"
  pi controller saturation/1 -> out/1
  Tappe/1 -> Add1/1
  Add2/1 -> pi controller saturation/1  "vdc_pi"
  Ki/1 -> Add1/2
  integral saturation/1 -> Add2/1, Tappe/1

== system general_charger_2 (Jordans MacBook.lan's conflicted copy 2013-12-22)/control_stage/AC//DC Control/DQ Controller/AB-DQ Transform/PLL/AB->DQ/Vq Discretization Error Correction/RMS4/PI3 ==
  in : Inport
  Add1 : Sum
  Add2 : Sum
  Ki : Gain  Gain=ki
  Kp : Gain  Gain=kp
  Tappe : simulink/Discrete/Tapped Delay  vinit=0.0  samptime=Ts_pi  NumDelays=1  DelayOrder=Oldest  includeCurrent=off
  Ts : Gain  Gain=Ts_pi
  integral saturation : Saturate  UpperLimit=int_sat_up  LowerLimit=int_sat_low  SampleTime=Ts_pi
  pi controller saturation : Saturate  UpperLimit=pi_sat_up  LowerLimit=pi_sat_low  SampleTime=Ts_pi
  out : Outport
  wires:
  Ts/1 -> Ki/1
  in/1 -> Kp/1, Ts/1  "vdc_error"
  Add1/1 -> integral saturation/1  "vdc_int_pi"
  Kp/1 -> Add2/2  "vdc_kp_pi"
  pi controller saturation/1 -> out/1
  Tappe/1 -> Add1/1
  Add2/1 -> pi controller saturation/1  "vdc_pi"
  Ki/1 -> Add1/2
  integral saturation/1 -> Add2/1, Tappe/1
